simulink library "BESS_lib"  (Simulink 8.1)
settings: Solver=ode45  SolverMode=SingleTasking  StartTime=0.0  StopTime=10.0  RelTol=1e-3
undefined symbols (not defined in the file or in its folder): DiscIntNeverNeededParam, gcbh, sps_rtmsupport, Ts
libraries: simulink x25, powerlib x6, powerlib_meascontrol x4, powerlib_extras x3, simulink_extras x1, debounce_lib x1
(part 1 of 2)
settings Model: Creator=ch24070  LastModifiedBy=hptb1  CovMetricSettings=dwe  CovHtmlReporting=off  covSaveCumulativeToWorkspaceVar=off  CovSaveSingleToWorkspaceVar=off  CovExternalEMLEnable=on

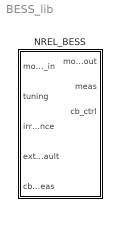
== system BESS_lib ==
  NREL_BESS : Subsystem  mask{InvType=ESS Inverter, Sn=250, Vn=480, b_Vdc_nom=1000, b_kWh=600, b_esr=0.1, r_I_max=3, Tc=Ts, MbusPrecInc=on, ExtTuningEna=on}
      mask prompts: InvType "Inverter type"; Sn "Nominal power [kVA]"; Vn "Nominal voltage ph-ph [V]"; b_Vdc_nom "Battery Vdc nominal [V]"; b_kWh "Battery capacity [kWh]"; b_esr "Battery ESR [Ohm]"; r_I_max "Max Current Ratio"; Tc "Control time step [s]"; MbusPrecInc "Increase power precision at Modbus interface (10x)"; ExtTuningEna "External tuning"
      mask init:
      | CFG.InvType = InvType;
      | CFG.Sn = Sn*1000;
      | CFG.Vn = Vn;
      | CFG.fn = 60;
      | CFG.r_I_max = r_I_max;
      | CFG.Tc = Tc;
      | 
      | if (MbusPrecInc == true)
      |     CFG.Prec = 10;
      | else
      |     CFG.Prec = 1;
      | end;
      | 
      | % get bess internal params (BP)
      | BP = BESS_init_mask(CFG);
      | 
      | 
      | dstr = 'Inverter data:\n';
      | dstr = [ dstr 'Sn=' num2str(Sn) 'kW\n'];
      | dstr = [ dstr 'Vn=' num2str(Vn/1000) 'kV\n'];
      | dstr = [ dstr 'In=' num2str(BP.In) 'A\n'];
      | dstr = [ dstr 'Imax=' num2str(BP.Imax) 'A\n'];
      mask TypeOptions InvType: PV Inverter | ESS Inverter
      mask Display: disp(dstr);

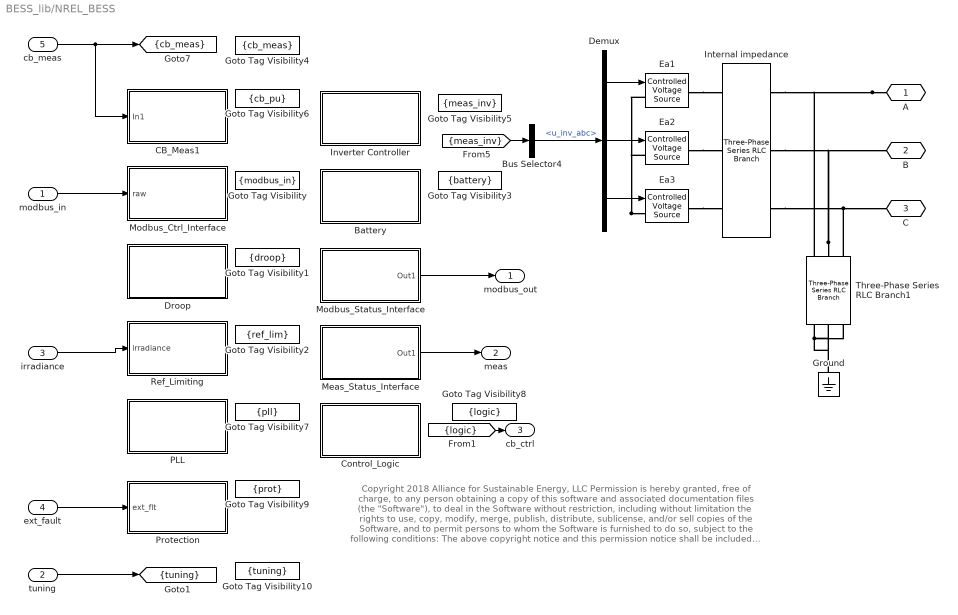
== system BESS_lib/NREL_BESS ==
  note: Copyright 2018 Alliance for Sustainable Energy, LLC
      |
      | Permission is hereby granted, free of charge, to any person obtaining a copy of this software
      | and associated documentation files (the "Software"), to deal in the Software without restriction,
      | including without limitation the rights to use, copy, modify, merge, publish, distribute, sublicense,
      | and/or sell copies of the Software, and to permit persons to whom the Software is furnished to do so,
      | subject to the following conditions:
      |
      | The above copyright notice and this permission notice shall be included in all copies or substantial portions of the Software.
      |
      | THE SOFTWARE IS PROVIDED "AS IS", WITHOUT WARRANTY OF ANY KIND, EXPRESS OR IMPLIED, INCLUDING
      | BUT NOT LIMITED TO THE WARRANTIES OF MERCHANTABILITY, FITNESS FOR A PARTICULAR PURPOSE AND
      | NONINFRINGEMENT. IN NO EVENT SHALL THE AUTHORS, THE COPYRIGHT HOLDERS, THE UNITED STATES,
      | THE UNITED STATES DEPARTMENT OF ENERGY, OR ANY OF THEIR EMPLOYEES BE LIABLE FOR ANY CLAIM,
      | DAMAGES OR OTHER LIABILITY, WHETHER IN AN ACTION OF CONTRACT, TORT OR OTHERWISE, ARISING FROM,
      | OUT OF OR IN CONNECTION WITH THE SOFTWARE OR THE USE OR OTHER DEALINGS IN THE SOFTWARE.
  modbus_in : Inport
  tuning : Inport  Port=2
  irradiance : Inport  Port=3
  ext_fault : Inport  Port=4
  cb_meas : Inport  Port=5
  Battery : Subsystem
  Bus Selector4 : BusSelector  OutputSignals=u_inv_abc
  CB_Meas1 : Subsystem
  Control_Logic : Subsystem
  Demux : Demux  Outputs=3
  Droop : Subsystem
  Ea1 : powerlib/Electrical Sources/Controlled Voltage Source  Initialize=off  Source_Type=DC  Amplitude=0  Phase=0  Frequency=0  Measurements=None
  Ea2 : powerlib/Electrical Sources/Controlled Voltage Source  Initialize=off  Source_Type=DC  Amplitude=0  Phase=0  Frequency=0  Measurements=None
  Ea3 : powerlib/Electrical Sources/Controlled Voltage Source  Initialize=off  Source_Type=DC  Amplitude=0  Phase=0  Frequency=0  Measurements=None
  Goto Tag Visibility : GotoTagVisibility  GotoTag=modbus_in
  Goto Tag Visibility1 : GotoTagVisibility  GotoTag=droop
  Goto Tag Visibility10 : GotoTagVisibility  GotoTag=tuning
  Goto Tag Visibility2 : GotoTagVisibility  GotoTag=ref_lim
  Goto Tag Visibility3 : GotoTagVisibility  GotoTag=battery
  Goto Tag Visibility4 : GotoTagVisibility  GotoTag=cb_meas
  Goto Tag Visibility5 : GotoTagVisibility  GotoTag=meas_inv
  Goto Tag Visibility6 : GotoTagVisibility  GotoTag=cb_pu
  Goto Tag Visibility7 : GotoTagVisibility  GotoTag=pll
  Goto Tag Visibility8 : GotoTagVisibility  GotoTag=logic
  Goto Tag Visibility9 : GotoTagVisibility  GotoTag=prot
  Ground : powerlib/Elements/Ground  LConnTagsString=a
  Internal impedance : powerlib/Elements/Three-Phase Series RLC Branch  LConnTagsString=A|B|C  RConnTagsString=A|B|C  BranchType=RL  Resistance=BP.R  Inductance=BP.L  Capacitance=1e-6  Measurements=None
  Inverter Controller : Subsystem
  Meas_Status_Interface : Subsystem
  Modbus_Ctrl_Interface : Subsystem
  Modbus_Status_Interface : Subsystem
  PLL : Subsystem
  Protection : Subsystem
  Ref_Limiting : Subsystem
  Three-Phase Series RLC Branch1 : powerlib/Elements/Three-Phase Series RLC Branch  LConnTagsString=A|B|C  RConnTagsString=A|B|C  BranchType=R  Resistance=10000  Inductance=1e-3  Capacitance=1000e-9  Measurements=None
  A : PMIOPort  Port=1  Side=Right
  B : PMIOPort  Port=2  Side=Right
  C : PMIOPort  Port=3  Side=Right
  modbus_out : Outport
  meas : Outport  Port=2
  cb_ctrl : Outport  Port=3
  tag scope: cb_meas=scoped, tuning=scoped
  wires:
  tuning/1 -> [tuning]
  ext_fault/1 -> Protection/1(ext_flt)
  Bus Selector4/1 -> Demux/1  "<u_inv_abc>"
  [meas_inv] -> Bus Selector4/1
  [logic] -> cb_ctrl/1
  Meas_Status_Interface/1(Out1) -> meas/1
  cb_meas/1 -> CB_Meas1/1(In1), [cb_meas]
  irradiance/1 -> Ref_Limiting/1(irradiance)
  Demux/1 -> Ea1/1
  Demux/2 -> Ea2/1
  Demux/3 -> Ea3/1
  Modbus_Status_Interface/1(Out1) -> modbus_out/1
  modbus_in/1 -> Modbus_Ctrl_Interface/1(raw)
  connections:
  Ea1/RConn1 -- Internal impedance/LConn1
  Ea2/RConn1 -- Internal impedance/LConn2
  Ea3/RConn1 -- Internal impedance/LConn3
  Ea3/LConn1 -- Ea2/LConn1 -- Ea1/LConn1
  A/RConn1 -- Internal impedance/RConn1 -- Three-Phase Series RLC Branch1/LConn1
  Internal impedance/RConn3 -- C/RConn1 -- Three-Phase Series RLC Branch1/LConn3
  Three-Phase Series RLC Branch1/LConn2 -- B/RConn1 -- Internal impedance/RConn2
  Three-Phase Series RLC Branch1/RConn1 -- Three-Phase Series RLC Branch1/RConn3 -- Three-Phase Series RLC Branch1/RConn2 -- Ground/LConn1

== system BESS_lib/NREL_BESS/Battery ==
  Battery : Subsystem  mask(Very simple battery model.){kWh=b_kWh, esr=b_esr, Vdc_nom=b_Vdc_nom}
      mask prompts: kWh "Capacity  (kWh)"; esr "Output Resistance (Ohms)"; Vdc_nom "Open Circuit Voltage"
      mask help: Model integrates charge and stops at the rated capacity. When charge is all removed the current drops to zero.
      mask Help: This model views the battery as a voltage source with a fixed equivalent series resistance and a perfect integrator for capacity.
  Bus Creator1 : BusCreator  Inputs=5
  Bus Selector1 : BusSelector  OutputSignals=batt_cap_div,batt_soc_rst
  Bus Selector4 : BusSelector  OutputSignals=relay_out.m.kw
  Compare To Constant : simulink/Logic and Bit Operations/Compare To Constant  relop===  const=1  OutDataTypeStr=boolean
  Compare To Constant1 : simulink/Logic and Bit Operations/Compare To Constant  relop===  const=-1  OutDataTypeStr=boolean
  Data Type Conversion : DataTypeConversion  OutDataTypeStr=double
  Data Type Conversion1 : DataTypeConversion  OutDataTypeStr=double
  Divide : Product  Inputs=*/
  Gain : Gain  Gain=100
  Gain2 : Gain  Gain=1000
  tag scope: battery=scoped
  wires:
  Bus Selector1/2 -> Battery/3(soc_rst)  "<batt_soc_rst>"
  Bus Selector1/1 -> Battery/2(cap_div)  "<batt_cap_div>"
  [tuning] -> Bus Selector1/1
  Gain2/1 -> Divide/1
  Bus Selector4/1 -> Gain2/1  "<kw>"
  Divide/1 -> Battery/1(Iout), Bus Creator1/5  "Idc"
  Battery/1(Vout) -> Bus Creator1/1, Divide/2  "Vdc"
  Gain/1 -> Bus Creator1/2  "SoC"
  Battery/2(Capacity) -> Gain/1
  Compare To Constant/1 -> Data Type Conversion/1
  Battery/3(Saturation) -> Compare To Constant1/1, Compare To Constant/1
  Compare To Constant1/1 -> Data Type Conversion1/1
  Bus Creator1/1 -> [battery]  "Battery"
  [cb_meas] -> Bus Selector4/1
  Data Type Conversion/1 -> Bus Creator1/3  "BattFull"
  Data Type Conversion1/1 -> Bus Creator1/4  "BattEmpty"

== system BESS_lib/NREL_BESS/CB_Meas1 ==
  In1 : Inport
  Bus Creator : BusCreator  Inputs=2
  Bus Selector : BusSelector  OutputSignals=cb_meas
  Bus Selector1 : BusSelector  OutputSignals=Vabc_line,Iabc
  Gain2 : Gain  Gain=1/BP.In/sqrt(2)
  Gain4 : Gain  Gain=1/(Vn*sqrt(2/3))
  tag scope: cb_pu=scoped
  wires:
  Bus Creator/1 -> [cb_pu]
  Gain2/1 -> Bus Creator/2  "iabc"
  Bus Selector1/2 -> Gain2/1  "<Iabc>"
  Gain4/1 -> Bus Creator/1  "vabc_line"
  Bus Selector1/1 -> Gain4/1  "<Vabc_line>"
  In1/1 -> Bus Selector/1
  Bus Selector/1 -> Bus Selector1/1  "<cb_meas>"

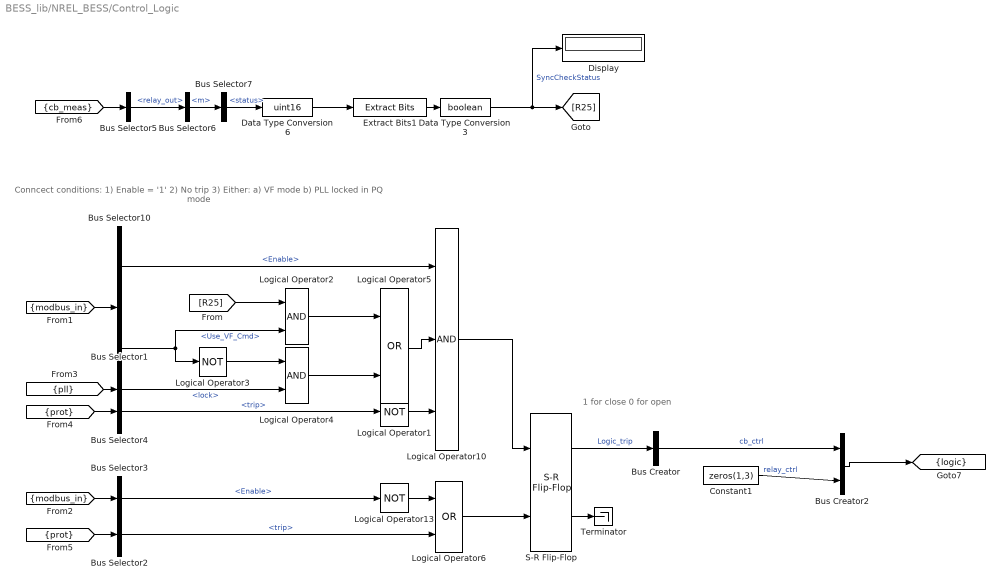
== system BESS_lib/NREL_BESS/Control_Logic ==
  note: 1 for close
      | 0 for open
  note: Conncect conditions:
      | 1) Enable = '1'
      | 2) No trip
      | 3) Either:
      | a) VF mode
      | b) PLL locked in PQ mode
  Bus Creator : BusCreator  Inputs=1
  Bus Creator2 : BusCreator  Inputs=2
  Bus Selector1 : BusSelector  OutputSignals=lock
  Bus Selector10 : BusSelector  OutputSignals=Control_Word.Enable,Control_Word.Use_VF_Cmd
  Bus Selector2 : BusSelector  OutputSignals=trip
  Bus Selector3 : BusSelector  OutputSignals=Control_Word.Enable
  Bus Selector4 : BusSelector  OutputSignals=trip
  Bus Selector5 : BusSelector  OutputSignals=relay_out
  Bus Selector6 : BusSelector  OutputSignals=m
  Bus Selector7 : BusSelector  OutputSignals=status
  Constant1 : Constant  Value=zeros(1,3)
  Data Type Conversion3 : DataTypeConversion  OutDataTypeStr=boolean
  Data Type Conversion6 : DataTypeConversion  OutDataTypeStr=uint16
  Display : Display
  Extract Bits1 : simulink/Logic and Bit Operations/Extract Bits  bitsToExtract=Range of bits  numBits=8  bitIdxRange=1  outScalingMode=Treat bit field as an integer
  Logical Operator1 : Logic  Operator=NOT  AllPortsSameDT=off  OutDataTypeStr=boolean
  Logical Operator10 : Logic  Inputs=3  AllPortsSameDT=off  OutDataTypeStr=boolean
  Logical Operator13 : Logic  Operator=NOT  AllPortsSameDT=off  OutDataTypeStr=boolean
  Logical Operator2 : Logic  AllPortsSameDT=off  OutDataTypeStr=boolean
  Logical Operator3 : Logic  Operator=NOT  AllPortsSameDT=off  OutDataTypeStr=boolean
  Logical Operator4 : Logic  AllPortsSameDT=off  OutDataTypeStr=boolean
  Logical Operator5 : Logic  Operator=OR  AllPortsSameDT=off  OutDataTypeStr=boolean
  Logical Operator6 : Logic  Operator=OR  AllPortsSameDT=off  OutDataTypeStr=boolean
  S-R Flip-Flop : simulink_extras/Flip Flops/S-R Flip-Flop  initial_condition=0
  Terminator : Terminator
  tag scope: logic=scoped
  wires:
  [R25] -> Logical Operator2/1
  Data Type Conversion3/1 -> [R25], Display/1  "SyncCheckStatus"
  Data Type Conversion6/1 -> Extract Bits1/1
  Extract Bits1/1 -> Data Type Conversion3/1
  Bus Selector7/1 -> Data Type Conversion6/1  "<status>"
  Bus Selector6/1 -> Bus Selector7/1  "<m>"
  Bus Selector5/1 -> Bus Selector6/1  "<relay_out>"
  [cb_meas] -> Bus Selector5/1
  Logical Operator2/1 -> Logical Operator5/1
  [prot] -> Bus Selector4/1
  Bus Selector4/1 -> Logical Operator1/1  "<trip>"
  [prot] -> Bus Selector2/1
  S-R Flip-Flop/2 -> Terminator/1
  Logical Operator13/1 -> Logical Operator6/1
  Bus Selector2/1 -> Logical Operator6/2  "<trip>"
  Logical Operator6/1 -> S-R Flip-Flop/2
  [modbus_in] -> Bus Selector3/1
  Bus Selector3/1 -> Logical Operator13/1  "<Enable>"
  Logical Operator1/1 -> Logical Operator10/3
  Logical Operator10/1 -> S-R Flip-Flop/1
  Logical Operator5/1 -> Logical Operator10/2
  Bus Selector1/1 -> Logical Operator4/2  "<lock>"
  Bus Selector10/2 -> Logical Operator3/1, Logical Operator2/2  "<Use_VF_Cmd>"
  [modbus_in] -> Bus Selector10/1
  Bus Selector10/1 -> Logical Operator10/1  "<Enable>"
  Constant1/1 -> Bus Creator2/2  "relay_ctrl"
  Bus Creator2/1 -> [logic]
  Bus Creator/1 -> Bus Creator2/1  "cb_ctrl"
  Logical Operator3/1 -> Logical Operator4/1
  [pll] -> Bus Selector1/1
  S-R Flip-Flop/1 -> Bus Creator/1  "Logic_trip"
  Logical Operator4/1 -> Logical Operator5/2

== system BESS_lib/NREL_BESS/Droop ==
  Bus Selector1 : BusSelector  OutputSignals=relay_out
  Bus Selector3 : BusSelector  OutputSignals=m.Hz,m.Va_rms,m.kw,m.kvar  OutputAsBus=on
  Bus Selector9 : BusSelector  OutputSignals=f_cmd,v_cmd,p_cmd,q_cmd  OutputAsBus=on
  Constant : Constant  Value=[0 0]
  Divide1 : Product  Inputs=*/
  Droop : Subsystem
  ExtractCoefs : Subsystem
  Mux1 : Mux  Inputs=2
  ScalingFactors1 : Constant  Value=[60 Vn/sqrt(3) [1 1]*Sn]
  Selector1 : Selector  InputPortWidth=4  IndexOptions=Index vector (dialog)  Indices=[1 2]  OutputSizes=1
  Sum1 : Sum  Inputs=-+|
  Sum2 : Sum  Inputs=++|
  tag scope: droop=scoped
  wires:
  ExtractCoefs/1(Out1) -> Droop/2(droop)
  [modbus_in] -> ExtractCoefs/1(In1)
  Bus Selector3/1 -> Divide1/1
  Bus Selector1/1 -> Bus Selector3/1  "<relay_out>"
  [cb_meas] -> Bus Selector1/1
  Bus Selector9/1 -> Selector1/1, Sum2/2
  [modbus_in] -> Bus Selector9/1
  Droop/1(dFvpq_out) -> Sum2/1
  Sum1/1 -> Droop/1(dfvpq)
  Selector1/1 -> Mux1/1
  Mux1/1 -> Sum1/2
  Constant/1 -> Mux1/2
  ScalingFactors1/1 -> Divide1/2
  Divide1/1 -> Sum1/1
  Sum2/1 -> [droop]

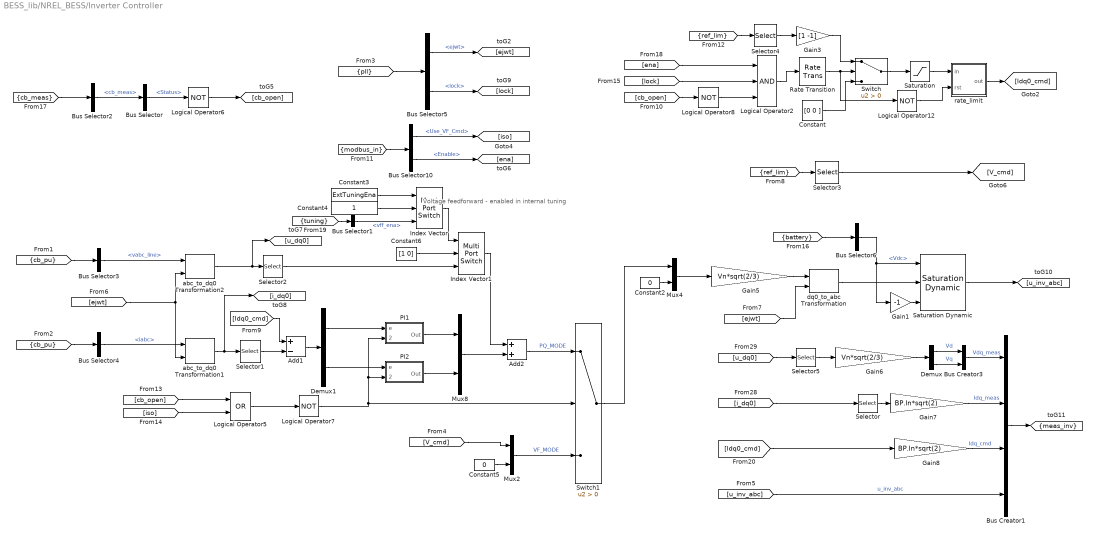
== system BESS_lib/NREL_BESS/Inverter Controller ==
  note: Voltage feedforward
      | - enabled in internal tuning
  Add1 : Sum  Inputs=+-
  Add2 : Sum
  Bus Creator1 : BusCreator
  Bus Creator3 : BusCreator  Inputs=2
  Bus Selector : BusSelector  OutputSignals=Status
  Bus Selector1 : BusSelector  OutputSignals=vff_ena
  Bus Selector10 : BusSelector  OutputSignals=Control_Word.Use_VF_Cmd,Control_Word.Enable
  Bus Selector2 : BusSelector  OutputSignals=cb_meas
  Bus Selector3 : BusSelector  OutputSignals=vabc_line
  Bus Selector4 : BusSelector  OutputSignals=iabc
  Bus Selector5 : BusSelector  OutputSignals=ejwt,lock
  Bus Selector6 : BusSelector  OutputSignals=Vdc
  Constant : Constant  Value=[0 0 ]
  Constant2 : Constant  Value=0
  Constant3 : Constant  Value=ExtTuningEna
  Constant4 : Constant
  Constant5 : Constant  Value=0
  Constant6 : Constant  Value=[1 0]
  Demux : Demux  Outputs=2
  Demux1 : Demux  Outputs=2
  Gain1 : Gain  Gain=-1
  Gain3 : Gain  Gain=[1 -1]
  Gain5 : Gain  Gain=Vn*sqrt(2/3)
  Gain6 : Gain  Gain=Vn*sqrt(2/3)
  Gain7 : Gain  Gain=BP.In*sqrt(2)
  Gain8 : Gain  Gain=BP.In*sqrt(2)
  Index Vector : MultiPortSwitch  DataPortOrder=Zero-based contiguous  Inputs=2  zeroidx=on
  Index Vector1 : MultiPortSwitch  DataPortOrder=Zero-based contiguous  Inputs=2  zeroidx=on
  Logical Operator{6..8,12} (4 alike) : Logic  Operator=NOT  AllPortsSameDT=off  OutDataTypeStr=boolean
  Logical Operator2 : Logic  Inputs=3  AllPortsSameDT=off  OutDataTypeStr=boolean
  Logical Operator5 : Logic  Operator=OR  AllPortsSameDT=off  OutDataTypeStr=boolean
  Mux2 : Mux  Inputs=2
  Mux4 : Mux  Inputs=[2 1]
  Mux8 : Mux  Inputs=2
  PI1 : Subsystem  mask{Kp=2, Ti=0.6e-3, Ts=Ts, D=0, Iup=1, Idown=-1, PIup=1, PIdown=-1, Int_init=0, Enable_zero_val=0}
      mask prompts: Kp "Proportional gain Kp"; Ti "Integral doubling-time Ti [s]"; Ts "Sample time [s]"; D "Derivative Gain"; Iup "Integral upper saturation limit"; Idown "Integral lower saturation limit"; PIup "PI output upper saturation limit"; PIdown "PI output lower saturation limit"; Int_init "Integral initial value"; Enable_zero_val "Output value when Enable=0"
      mask help: PID controller integral is in enable state when Enable signal value equals 1. If Enable state equals zero the PID output also equals zero.
  PI2 : Subsystem  mask{Kp=2, Ti=0.6e-3, Ts=Ts, D=0, Iup=1, Idown=-1, PIup=1, PIdown=-1, Int_init=0, Enable_zero_val=0}
      mask prompts: Kp "Proportional gain Kp"; Ti "Integral doubling-time Ti [s]"; Ts "Sample time [s]"; D "Derivative Gain"; Iup "Integral upper saturation limit"; Idown "Integral lower saturation limit"; PIup "PI output upper saturation limit"; PIdown "PI output lower saturation limit"; Int_init "Integral initial value"; Enable_zero_val "Output value when Enable=0"
      mask help: PID controller integral is in enable state when Enable signal value equals 1. If Enable state equals zero the PID output also equals zero.
  Rate Transition : RateTransition  OutPortSampleTime=Tc
  Saturation : Saturate  UpperLimit=BP.Imax*sqrt(2)  LowerLimit=-BP.Imax*sqrt(2)
  Saturation Dynamic : simulink/Discontinuities/Saturation Dynamic  OutMin=[]  OutMax=[]  OutDataTypeStr=Inherit: Same as second input  OutDataType=fixdt(1, 16)  OutScaling=2^-10  DoSatur=off
  Selector{,1..2,5} (4 alike) : Selector  InputPortWidth=3  IndexOptions=Index vector (dialog)  Indices=[1 2]  OutputSizes=1
  Selector3 : Selector  InputPortWidth=4  IndexOptions=Index vector (dialog)  Indices=2  OutputSizes=1
  Selector4 : Selector  InputPortWidth=4  IndexOptions=Index vector (dialog)  Indices=[3 4]  OutputSizes=1
  Switch : Switch  Criteria=u2 > Threshold
  Switch1 : Switch  Criteria=u2 > Threshold
  abc_to_dq0 Transformation1 : powerlib_extras/Measurements/abc_to_dq0 Transformation
  abc_to_dq0 Transformation2 : powerlib_extras/Measurements/abc_to_dq0 Transformation
  dq0_to_abc Transformation : powerlib_extras/Measurements/dq0_to_abc Transformation
  rate_limit : Subsystem
  tag scope: meas_inv=scoped
  wires:
  Constant6/1 -> Index Vector1/2
  Selector2/1 -> Index Vector1/3
  Index Vector/1 -> Index Vector1/1
  Constant4/1 -> Index Vector/2
  Bus Selector1/1 -> Index Vector/3  "<vff_ena>"
  [tuning] -> Bus Selector1/1
  Constant3/1 -> Index Vector/1
  Bus Selector6/1 -> Gain1/1, Saturation Dynamic/1  "<Vdc>"
  [battery] -> Bus Selector6/1
  Bus Selector10/1 -> [iso]  "<Use_VF_Cmd>"
  [modbus_in] -> Bus Selector10/1
  Bus Selector10/2 -> [ena]  "<Enable>"
  [ref_lim] -> Selector3/1
  [ref_lim] -> Selector4/1
  [u_inv_abc] -> Bus Creator1/4  "u_inv_abc"
  Bus Selector5/2 -> [lock]  "<lock>"
  Bus Selector5/1 -> [ejwt]  "<ejwt>"
  [pll] -> Bus Selector5/1
  [cb_pu] -> Bus Selector4/1
  [cb_pu] -> Bus Selector3/1
  Gain3/1 -> Switch/1
  Bus Selector2/1 -> Bus Selector/1  "<cb_meas>"
  Demux/2 -> Bus Creator3/2  "Vq"
  Demux/1 -> Bus Creator3/1  "Vd"
  Gain6/1 -> Demux/1
  Bus Creator3/1 -> Bus Creator1/1  "Vdq_meas"
  Gain8/1 -> Bus Creator1/3  "Idq_cmd"
  Gain7/1 -> Bus Creator1/2  "Idq_meas"
  Gain5/1 -> dq0_to_abc Transformation/1
  Bus Selector3/1 -> abc_to_dq0 Transformation2/1  "<vabc_line>"
  Bus Selector4/1 -> abc_to_dq0 Transformation1/1  "<iabc>"
  Gain1/1 -> Saturation Dynamic/3
  Saturation Dynamic/1 -> [u_inv_abc]
  Logical Operator12/1 -> rate_limit/2(rst)
  rate_limit/1(out) -> [Idq0_cmd]
  Selector5/1 -> Gain6/1
  Constant2/1 -> Mux4/2
  Mux4/1 -> Gain5/1
  Switch1/1 -> Mux4/1
  Index Vector1/1 -> Add2/1
  Selector1/1 -> Add1/2
  [i_dq0] -> Selector/1
  Bus Creator1/1 -> [meas_inv]
  [u_dq0] -> Selector5/1
  [Idq0_cmd] -> Gain8/1
  Selector/1 -> Gain7/1
  Selector3/1 -> [V_cmd]
  [ena] -> Logical Operator2/1
  Add2/1 -> Switch1/1  "PQ_MODE"
  Mux8/1 -> Add2/2
  abc_to_dq0 Transformation2/1 -> Selector2/1, [u_dq0]
  [lock] -> Logical Operator2/2
  [Idq0_cmd] -> Add1/1
  Saturation/1 -> rate_limit/1(in)
  Logical Operator8/1 -> Logical Operator2/3
  [cb_open] -> Logical Operator8/1
  [cb_open] -> Logical Operator5/1
  Logical Operator6/1 -> [cb_open]
  Bus Selector/1 -> Logical Operator6/1  "<Status>"
  [iso] -> Logical Operator5/2
  Logical Operator7/1 -> PI1/2(Enable), PI2/2(Enable), Switch1/2
  Logical Operator2/1 -> Rate Transition/1
  Constant/1 -> Switch/3
  Switch/1 -> Saturation/1
  Rate Transition/1 -> Switch/2, Logical Operator12/1
  Add1/1 -> Demux1/1
  Demux1/2 -> PI2/1(e)
  Demux1/1 -> PI1/1(e)
  Mux2/1 -> Switch1/3  "VF_MODE"
  Constant5/1 -> Mux2/2
  [V_cmd] -> Mux2/1
  Logical Operator5/1 -> Logical Operator7/1
  PI2/1(Out) -> Mux8/2
  PI1/1(Out) -> Mux8/1
  [ejwt] -> abc_to_dq0 Transformation2/2, abc_to_dq0 Transformation1/2
  [ejwt] -> dq0_to_abc Transformation/2
  Selector4/1 -> Gain3/1
  abc_to_dq0 Transformation1/1 -> Selector1/1, [i_dq0]
  [cb_meas] -> Bus Selector2/1
  dq0_to_abc Transformation/1 -> Saturation Dynamic/2

== system BESS_lib/NREL_BESS/Meas_Status_Interface ==
  Bus Creator4 : BusCreator  Inputs=6
  Bus Selector1 : BusSelector  OutputSignals=cb_ctrl.Logic_trip
  Bus Selector2 : BusSelector  OutputSignals=raw
  Bus Selector4 : BusSelector  OutputSignals=status,flt_word  OutputAsBus=on
  Data Type Conversion : DataTypeConversion  OutDataTypeStr=double
  Gain : Gain  Gain=[1 8]
  Sum : Sum  Inputs=+
  Out1 : Outport
  wires:
  Bus Selector2/1 -> Bus Creator4/6  "<raw>"
  [modbus_in] -> Bus Selector2/1
  Data Type Conversion/1 -> Bus Creator4/5  "Logic_trip"
  Bus Selector1/1 -> Data Type Conversion/1  "<Logic_trip>"
  [logic] -> Bus Selector1/1
  Sum/1 -> Bus Creator4/4  "status_word"
  Gain/1 -> Sum/1
  Bus Selector4/1 -> Gain/1
  [prot] -> Bus Selector4/1
  [meas_inv] -> Bus Creator4/1  "Inverter"
  [cb_meas] -> Bus Creator4/2  "CB_meas"
  Bus Creator4/1 -> Out1/1
  [battery] -> Bus Creator4/3  "Battery"

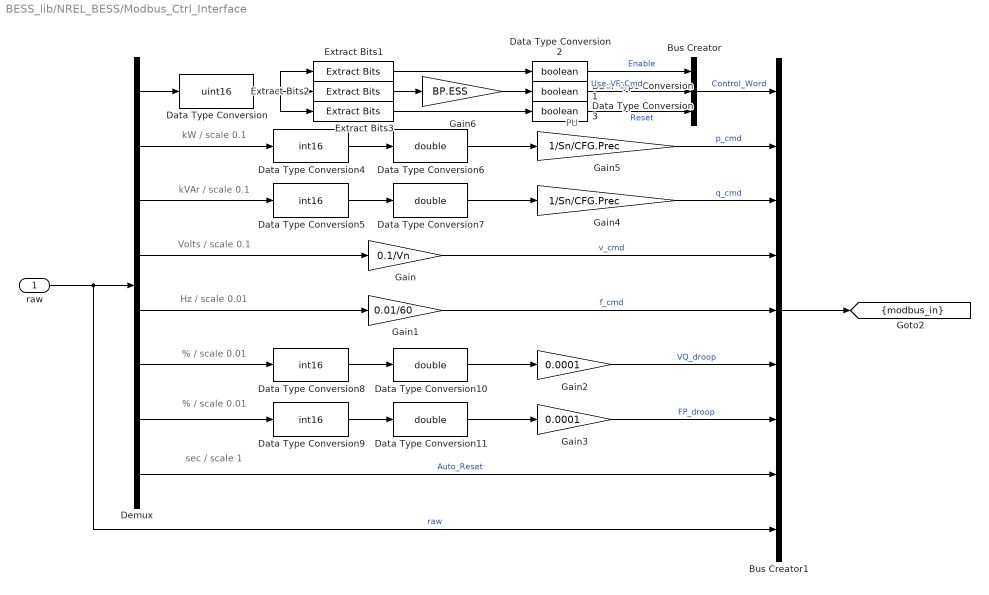
== system BESS_lib/NREL_BESS/Modbus_Ctrl_Interface ==
  note: sec / scale 1
  note: % / scale 0.01
  note: % / scale 0.01
  note: Hz / scale 0.01
  note: Volts / scale 0.1
  note: kVAr / scale 0.1
  note: PU
  note: kW / scale 0.1
  raw : Inport
  Bus Creator : BusCreator  Inputs=3
  Bus Creator1 : BusCreator  Inputs=9
  Data Type Conversion : DataTypeConversion  OutDataTypeStr=uint16
  Data Type Conversion1 : DataTypeConversion  OutDataTypeStr=boolean
  Data Type Conversion{6..7,10..11} (4 alike) : DataTypeConversion  OutDataTypeStr=double
  Data Type Conversion2 : DataTypeConversion  OutDataTypeStr=boolean
  Data Type Conversion3 : DataTypeConversion  OutDataTypeStr=boolean
  Data Type Conversion{4..5,8..9} (4 alike) : DataTypeConversion  OutDataTypeStr=int16
  Demux : Demux  Outputs=8
  Extract Bits1 : simulink/Logic and Bit Operations/Extract Bits  bitsToExtract=Range of bits  numBits=8  bitIdxRange=[0]  outScalingMode=Treat bit field as an integer
  Extract Bits2 : simulink/Logic and Bit Operations/Extract Bits  bitsToExtract=Range of bits  numBits=8  bitIdxRange=[1]  outScalingMode=Treat bit field as an integer
  Extract Bits3 : simulink/Logic and Bit Operations/Extract Bits  bitsToExtract=Range of bits  numBits=8  bitIdxRange=[2]  outScalingMode=Treat bit field as an integer
  Gain : Gain  Gain=0.1/Vn
  Gain1 : Gain  Gain=0.01/60
  Gain2 : Gain  Gain=0.0001
  Gain3 : Gain  Gain=0.0001
  Gain4 : Gain  Gain=1/Sn/CFG.Prec
  Gain5 : Gain  Gain=1/Sn/CFG.Prec
  Gain6 : Gain  Gain=BP.ESS
  tag scope: modbus_in=scoped
  wires:
  raw/1 -> Demux/1, Bus Creator1/9  "raw"
  Data Type Conversion11/1 -> Gain3/1
  Data Type Conversion10/1 -> Gain2/1
  Data Type Conversion9/1 -> Data Type Conversion11/1
  Data Type Conversion8/1 -> Data Type Conversion10/1
  Gain6/1 -> Data Type Conversion1/1
  Data Type Conversion7/1 -> Gain4/1
  Data Type Conversion6/1 -> Gain5/1
  Data Type Conversion5/1 -> Data Type Conversion7/1
  Data Type Conversion4/1 -> Data Type Conversion6/1
  Gain5/1 -> Bus Creator1/2  "p_cmd"
  Gain4/1 -> Bus Creator1/3  "q_cmd"
  Demux/2 -> Data Type Conversion4/1
  Data Type Conversion3/1 -> Bus Creator/3  "Reset"
  Data Type Conversion1/1 -> Bus Creator/2  "Use_VF_Cmd"
  Data Type Conversion2/1 -> Bus Creator/1  "Enable"
  Bus Creator1/1 -> [modbus_in]
  Demux/8 -> Bus Creator1/8  "Auto_Reset"
  Gain3/1 -> Bus Creator1/7  "FP_droop"
  Demux/7 -> Data Type Conversion9/1
  Gain2/1 -> Bus Creator1/6  "VQ_droop"
  Demux/6 -> Data Type Conversion8/1
  Gain1/1 -> Bus Creator1/5  "f_cmd"
  Demux/5 -> Gain1/1
  Gain/1 -> Bus Creator1/4  "v_cmd"
  Demux/4 -> Gain/1
  Demux/3 -> Data Type Conversion5/1
  Bus Creator/1 -> Bus Creator1/1  "Control_Word"
  Extract Bits3/1 -> Data Type Conversion3/1
  Extract Bits2/1 -> Gain6/1
  Extract Bits1/1 -> Data Type Conversion2/1
  Data Type Conversion/1 -> Extract Bits1/1, Extract Bits2/1, Extract Bits3/1
  Demux/1 -> Data Type Conversion/1

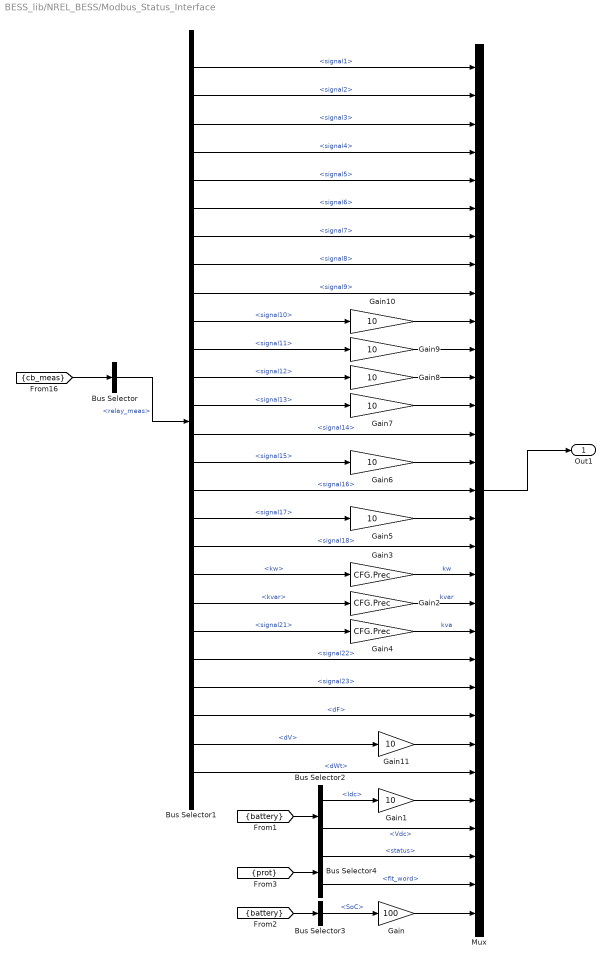
== system BESS_lib/NREL_BESS/Modbus_Status_Interface ==
  Bus Selector : BusSelector  OutputSignals=relay_meas
  Bus Selector1 : BusSelector  OutputSignals=signal1,signal2,signal3,signal4,signal5,signal6,signal7,signal8,signal9,signal10,signal11,signal12,signal13,signal14,signal15,signal16,signal17,signal18,kw,kvar,signal21,signal22,signal23,dF,dV,dWt
  Bus Selector2 : BusSelector  OutputSignals=Idc,Vdc
  Bus Selector3 : BusSelector  OutputSignals=SoC
  Bus Selector4 : BusSelector  OutputSignals=status,flt_word
  Gain : Gain  Gain=100
  Gain{1,5..11} (8 alike) : Gain  Gain=10
  Gain2 : Gain  Gain=CFG.Prec
  Gain3 : Gain  Gain=CFG.Prec
  Gain4 : Gain  Gain=CFG.Prec
  Mux : Mux  Inputs=31
  Out1 : Outport
  wires:
  Gain11/1 -> Mux/25
  Bus Selector1/26 -> Mux/26  "<dWt>"
  Bus Selector1/25 -> Gain11/1  "<dV>"
  Bus Selector1/24 -> Mux/24  "<dF>"
  Gain10/1 -> Mux/10
  Gain9/1 -> Mux/11
  Gain8/1 -> Mux/12
  Gain7/1 -> Mux/13
  Gain6/1 -> Mux/15
  Gain5/1 -> Mux/17
  Gain3/1 -> Mux/19  "kw"
  Gain2/1 -> Mux/20  "kvar"
  Gain4/1 -> Mux/21  "kva"
  Bus Selector4/1 -> Mux/29  "<status>"
  [prot] -> Bus Selector4/1
  Gain1/1 -> Mux/27
  Gain/1 -> Mux/31
  Bus Selector4/2 -> Mux/30  "<flt_word>"
  Bus Selector3/1 -> Gain/1  "<SoC>"
  [battery] -> Bus Selector3/1
  Bus Selector2/1 -> Gain1/1  "<Idc>"
  Bus Selector2/2 -> Mux/28  "<Vdc>"
  [battery] -> Bus Selector2/1
  Bus Selector1/23 -> Mux/23  "<signal23>"
  Bus Selector1/22 -> Mux/22  "<signal22>"
  Bus Selector1/21 -> Gain4/1  "<signal21>"
  Bus Selector1/20 -> Gain2/1  "<kvar>"
  Bus Selector1/19 -> Gain3/1  "<kw>"
  Bus Selector1/18 -> Mux/18  "<signal18>"
  Bus Selector1/17 -> Gain5/1  "<signal17>"
  Bus Selector1/16 -> Mux/16  "<signal16>"
  Bus Selector1/15 -> Gain6/1  "<signal15>"
  Bus Selector1/14 -> Mux/14  "<signal14>"
  Bus Selector1/13 -> Gain7/1  "<signal13>"
  Bus Selector1/12 -> Gain8/1  "<signal12>"
  Bus Selector1/11 -> Gain9/1  "<signal11>"
  Bus Selector1/10 -> Gain10/1  "<signal10>"
  Bus Selector1/9 -> Mux/9  "<signal9>"
  Bus Selector1/8 -> Mux/8  "<signal8>"
  Bus Selector1/7 -> Mux/7  "<signal7>"
  Bus Selector1/6 -> Mux/6  "<signal6>"
  Bus Selector1/5 -> Mux/5  "<signal5>"
  Bus Selector1/4 -> Mux/4  "<signal4>"
  Bus Selector1/3 -> Mux/3  "<signal3>"
  Bus Selector1/2 -> Mux/2  "<signal2>"
  Bus Selector1/1 -> Mux/1  "<signal1>"
  Bus Selector/1 -> Bus Selector1/1  "<relay_meas>"
  Mux/1 -> Out1/1
  [cb_meas] -> Bus Selector/1

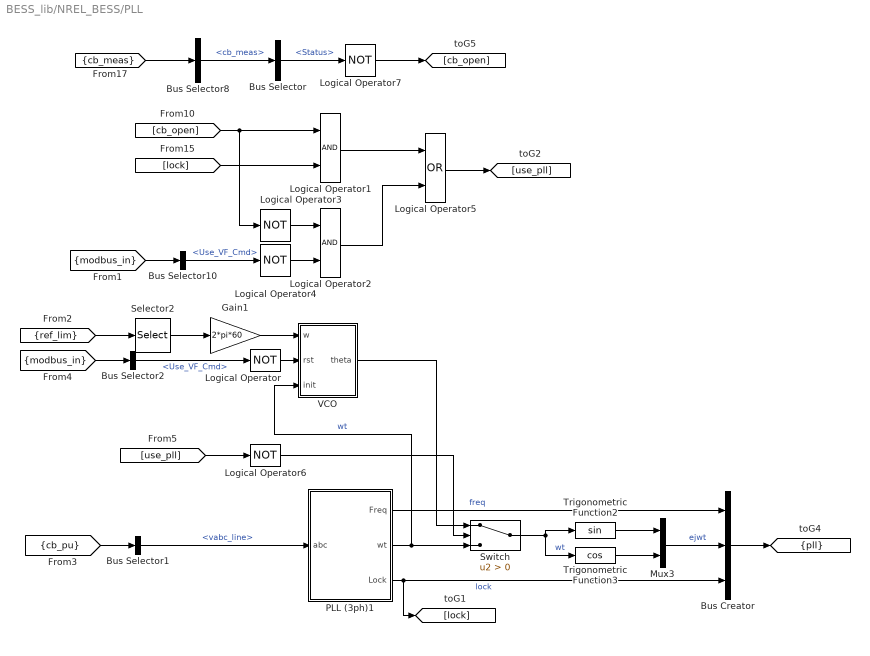
== system BESS_lib/NREL_BESS/PLL ==
  Bus Creator : BusCreator  Inputs=3
  Bus Selector : BusSelector  OutputSignals=Status
  Bus Selector1 : BusSelector  OutputSignals=vabc_line
  Bus Selector10 : BusSelector  OutputSignals=Control_Word.Use_VF_Cmd
  Bus Selector2 : BusSelector  OutputSignals=Control_Word.Use_VF_Cmd
  Bus Selector8 : BusSelector  OutputSignals=cb_meas
  Gain1 : Gain  Gain=2*pi*60  SaturateOnIntegerOverflow=on  OutDataTypeStr=Inherit: Same as input  ParamDataTypeStr=Inherit: Same as input
  Logical Operator{,3..4,6..7} (5 alike) : Logic  Operator=NOT  AllPortsSameDT=off  OutDataTypeStr=boolean
  Logical Operator1 : Logic  AllPortsSameDT=off  OutDataTypeStr=boolean
  Logical Operator2 : Logic  AllPortsSameDT=off  OutDataTypeStr=boolean
  Logical Operator5 : Logic  Operator=OR  AllPortsSameDT=off  OutDataTypeStr=boolean
  Mux3 : Mux  Inputs=2
  PLL (3ph)1 : Subsystem  DialogController=POWERSYS.PowerSysDialog  LoadFcn=sps_rtmsupport('LoadFcn', gcbh);  StartFcn=sps_rtmsupport('StartFcn', gcbh);  StopFcn=sps_rtmsupport('StopFcn', gcbh);  mask(PLL (3ph)){Flim=[55 66], Par_Init=[0, 60], ParK=[180, 3200, 1], TcD=Tc, MaxRateChangeFreq=12, FilterCutOffFreq=25, Ts=Tc, AGC=off}
      mask prompts: Flim "Minimum frequency (Hz):"; Par_Init "Initial inputs [ Phase (degrees), Frequency (Hz) ]:"; ParK "Regulator gains [ Kp, Ki, Kd ]:"; TcD "Time constant for derivative action (s):"; MaxRateChangeFreq "Maximum rate of change of frequency (Hz/s):"; FilterCutOffFreq "Filter cut-off frequency for frequency measurement (Hz):"; Ts "Sample time:"; AGC "Enable automatic gain control"
      mask help:
      | This Phase Locked Loop (PLL) system can be used  to synchronize on a set of variable frequency, three-phase sinusoidal signals. If the Automatic Gain Control is enabled, the input (phase error) of the PLL regulator is scaled according to the input signals magnitude.
      |
      | For optimal performance, set regulator gains [ Kp Ki  Kd ] = [ 180  3200  1 ] and check the Enable Automatic Gain Control parameter.
      |
      | Input : Vector containing the normalized three-phase signals [Va Vb Vc]
      | Output 1:  Measured frequency (Hz) = w/(2pi)
      | Output 2:  Ramp w.t varying between  0 and 2*pi, synchronized on zero crossings of the fundamental (positive-sequence) of phase A.
      mask init:
      | %block=gcb;
      | %[WantBlockChoice,Ts,sps] = powericon('PLL3phInit',block,Fmin,Par_Init,ParK,TcD, MaxRateChangeFreq, FilterCutOffFreq, AGC,Ts);
      | %powericon('SetInternalModels','set',block,WantBlockChoice);
      settings: CopyFcn=sps_rtmsupport('CopyFcn', gcbh);  DeleteFcn=sps_rtmsupport('DeleteFcn', gcbh);  UndoDeleteFcn=sps_rtmsupport('UndoDeleteFcn', gcbh);  ModelCloseFcn=sps_rtmsupport('ModelCloseFcn', gcbh);  PreSaveFcn=sps_rtmsupport('PreSaveFcn', gcbh);  PostSaveFcn=sps_rtmsupport('PostSaveFcn', gcbh);  NameChangeFcn=sps_rtmsupport('NameChangeFcn', gcbh);  PreCopyFcn=sps_rtmsupport('PreCopyFcn', gcbh);  CloseFcn=sps_rtmsupport('CloseFcn', gcbh);  PreDeleteFcn=sps_rtmsupport('PreDeleteFcn', gcbh);
      settings: OpenFcn=|
      | power_openblockproxy();
      | sps_rtmsupport('OpenFcn', gcbh, [8]);
      mask Help: helpview(psbhelp);
  Selector2 : Selector  InputPortWidth=4  IndexOptions=Index vector (dialog)  Indices=[1]  OutputSizes=1
  Switch : Switch  Criteria=u2 > Threshold
  Trigonometric Function2 : Trigonometry
  Trigonometric Function3 : Trigonometry  Operator=cos
  VCO : Subsystem
  tag scope: pll=scoped
  wires:
  Logical Operator6/1 -> Switch/2
  Logical Operator5/1 -> [use_pll]
  Logical Operator2/1 -> Logical Operator5/2
  Logical Operator4/1 -> Logical Operator2/2
  Logical Operator3/1 -> Logical Operator2/1
  Bus Selector10/1 -> Logical Operator4/1  "<Use_VF_Cmd>"
  Bus Selector2/1 -> Logical Operator/1  "<Use_VF_Cmd>"
  [modbus_in] -> Bus Selector2/1
  Logical Operator1/1 -> Logical Operator5/1
  [lock] -> Logical Operator1/2
  [cb_open] -> Logical Operator1/1, Logical Operator3/1
  Bus Selector8/1 -> Bus Selector/1  "<cb_meas>"
  Logical Operator7/1 -> [cb_open]
  Bus Selector/1 -> Logical Operator7/1  "<Status>"
  [cb_meas] -> Bus Selector8/1
  Logical Operator/1 -> VCO/2(rst)
  PLL (3ph)1/2(wt) -> Switch/3, VCO/3(init)  "wt"
  VCO/1(theta) -> Switch/1
  Gain1/1 -> VCO/1(w)
  [cb_pu] -> Bus Selector1/1
  [ref_lim] -> Selector2/1
  [use_pll] -> Logical Operator6/1
  [modbus_in] -> Bus Selector10/1
  Bus Creator/1 -> [pll]
  Selector2/1 -> Gain1/1
  PLL (3ph)1/1(Freq) -> Bus Creator/1  "freq"
  PLL (3ph)1/3(Lock) -> Bus Creator/3, [lock]  "lock"
  Bus Selector1/1 -> PLL (3ph)1/1(abc)  "<vabc_line>"
  Trigonometric Function3/1 -> Mux3/2
  Trigonometric Function2/1 -> Mux3/1
  Switch/1 -> Trigonometric Function3/1, Trigonometric Function2/1  "wt"
  Mux3/1 -> Bus Creator/2  "ejwt"

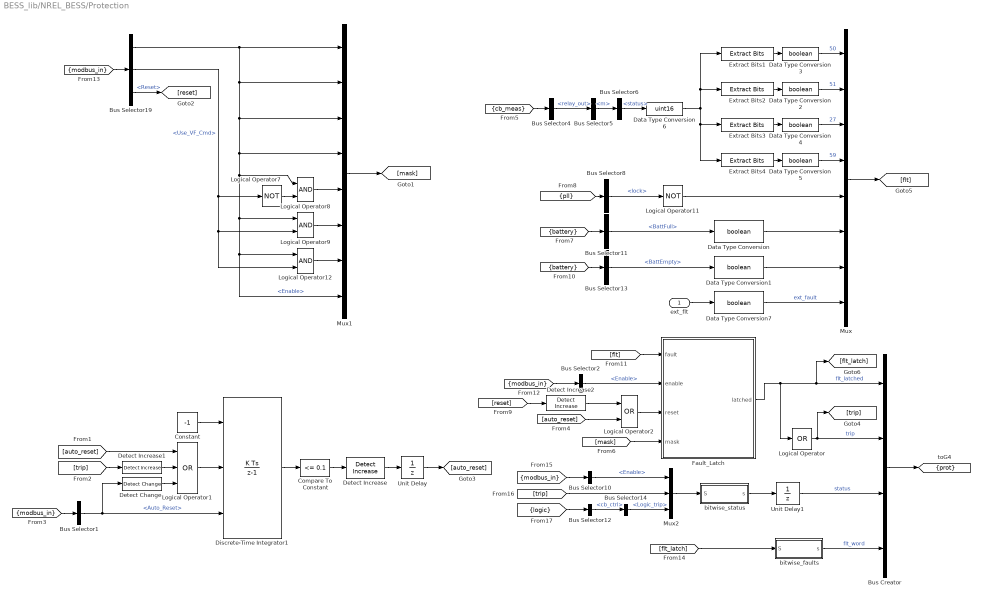
== system BESS_lib/NREL_BESS/Protection ==
  ext_flt : Inport
  Bus Creator : BusCreator
  Bus Selector1 : BusSelector  OutputSignals=Auto_Reset
  Bus Selector10 : BusSelector  OutputSignals=Control_Word.Enable
  Bus Selector11 : BusSelector  OutputSignals=BattFull
  Bus Selector12 : BusSelector  OutputSignals=cb_ctrl
  Bus Selector13 : BusSelector  OutputSignals=BattEmpty
  Bus Selector14 : BusSelector  OutputSignals=Logic_trip
  Bus Selector19 : BusSelector  OutputSignals=Control_Word.Enable,Control_Word.Use_VF_Cmd,Control_Word.Reset
  Bus Selector2 : BusSelector  OutputSignals=Control_Word.Enable
  Bus Selector4 : BusSelector  OutputSignals=relay_out
  Bus Selector5 : BusSelector  OutputSignals=m
  Bus Selector6 : BusSelector  OutputSignals=status
  Bus Selector8 : BusSelector  OutputSignals=lock
  Compare To Constant : simulink/Logic and Bit Operations/Compare To Constant  relop=<=  const=0.1  OutDataTypeStr=boolean
  Constant : Constant  Value=-1
  Data Type Conversion{,1..5,7} (7 alike) : DataTypeConversion  OutDataTypeStr=boolean
  Data Type Conversion6 : DataTypeConversion  OutDataTypeStr=uint16
  Detect Change : simulink/Logic and Bit Operations/Detect Change  vinit=0  InputProcessing=Inherited  OutDataTypeStr=boolean
  Detect Increase : simulink/Logic and Bit Operations/Detect Increase  vinit=0.0  InputProcessing=Inherited  OutDataTypeStr=boolean
  Detect Increase1 : simulink/Logic and Bit Operations/Detect Increase  vinit=0.0  InputProcessing=Inherited  OutDataTypeStr=boolean
  Detect Increase2 : simulink/Logic and Bit Operations/Detect Increase  vinit=0.0  InputProcessing=Inherited  OutDataTypeStr=boolean
  Discrete-Time Integrator1 : DiscreteIntegrator  ExternalReset=rising  InitialConditionSource=external  SampleTime=Ts  LimitOutput=on  LowerSaturationLimit=0  ICPrevOutput=DiscIntNeverNeededParam  ICPrevScaledInput=DiscIntNeverNeededParam
  Extract Bits1 : simulink/Logic and Bit Operations/Extract Bits  bitsToExtract=Range of bits  numBits=8  bitIdxRange=7  outScalingMode=Treat bit field as an integer
  Extract Bits2 : simulink/Logic and Bit Operations/Extract Bits  bitsToExtract=Range of bits  numBits=8  bitIdxRange=8  outScalingMode=Treat bit field as an integer
  Extract Bits3 : simulink/Logic and Bit Operations/Extract Bits  bitsToExtract=Range of bits  numBits=8  bitIdxRange=9  outScalingMode=Treat bit field as an integer
  Extract Bits4 : simulink/Logic and Bit Operations/Extract Bits  bitsToExtract=Range of bits  numBits=8  bitIdxRange=10  outScalingMode=Treat bit field as an integer
  Fault_Latch : Subsystem
  Logical Operator : Logic  Operator=OR  Inputs=1  AllPortsSameDT=off  OutDataTypeStr=boolean
  Logical Operator1 : Logic  Operator=OR  Inputs=3  AllPortsSameDT=off  OutDataTypeStr=boolean
  Logical Operator11 : Logic  Operator=NOT  AllPortsSameDT=off  OutDataTypeStr=boolean
  Logical Operator12 : Logic  AllPortsSameDT=off  OutDataTypeStr=boolean
  Logical Operator2 : Logic  Operator=OR  AllPortsSameDT=off  OutDataTypeStr=boolean
  Logical Operator7 : Logic  Operator=NOT  AllPortsSameDT=off  OutDataTypeStr=boolean
  Logical Operator8 : Logic  AllPortsSameDT=off  OutDataTypeStr=boolean
  Logical Operator9 : Logic  AllPortsSameDT=off  OutDataTypeStr=boolean
  Mux : Mux  Inputs=8
  Mux1 : Mux  Inputs=8
  Mux2 : Mux  Inputs=3
  Unit Delay : UnitDelay  SampleTime=-1
  Unit Delay1 : UnitDelay  SampleTime=-1
  bitwise_faults : Subsystem
  bitwise_status : Subsystem
  tag scope: prot=scoped
  wires:
  Data Type Conversion7/1 -> Mux/8  "ext_fault"
  ext_flt/1 -> Data Type Conversion7/1
  Unit Delay1/1 -> Bus Creator/3  "status"
  Bus Selector14/1 -> Mux2/3  "<Logic_trip>"
  Bus Selector12/1 -> Bus Selector14/1  "<cb_ctrl>"
  [logic] -> Bus Selector12/1
  [trip] -> Mux2/2
  Bus Selector10/1 -> Mux2/1  "<Enable>"
  [modbus_in] -> Bus Selector10/1
  Mux2/1 -> bitwise_status/1(S)
  [flt_latch] -> bitwise_faults/1(S)
  bitwise_faults/1(s) -> Bus Creator/4  "flt_word"
  bitwise_status/1(s) -> Unit Delay1/1
  Detect Change/1 -> Logical Operator1/3
  [flt] -> Fault_Latch/1(fault)
  Mux/1 -> [flt]
  Detect Increase2/1 -> Logical Operator2/1
  [reset] -> Detect Increase2/1
  [auto_reset] -> Logical Operator2/2
  Logical Operator2/1 -> Fault_Latch/3(reset)
  Bus Selector1/1 -> Discrete-Time Integrator1/3, Detect Change/1  "<Auto_Reset>"
  [modbus_in] -> Bus Selector1/1
  Unit Delay/1 -> [auto_reset]
  Detect Increase/1 -> Unit Delay/1
  Logical Operator1/1 -> Discrete-Time Integrator1/2
  [auto_reset] -> Logical Operator1/1
  Detect Increase1/1 -> Logical Operator1/2
  Compare To Constant/1 -> Detect Increase/1
  Discrete-Time Integrator1/1 -> Compare To Constant/1
  [trip] -> Detect Increase1/1
  Constant/1 -> Discrete-Time Integrator1/1
  Bus Creator/1 -> [prot]
  Logical Operator/1 -> [trip], Bus Creator/2  "trip"
  Data Type Conversion6/1 -> Extract Bits1/1, Extract Bits2/1, Extract Bits4/1, Extract Bits3/1
  Data Type Conversion5/1 -> Mux/4  "59"
  Data Type Conversion4/1 -> Mux/3  "27"
  Data Type Conversion2/1 -> Mux/2  "51"
  Data Type Conversion3/1 -> Mux/1  "50"
  Data Type Conversion1/1 -> Mux/7
  Data Type Conversion/1 -> Mux/6
  Fault_Latch/1(latched) -> Bus Creator/1, [flt_latch], Logical Operator/1  "flt_latched"
  Bus Selector19/3 -> [reset]  "<Reset>"
  [mask] -> Fault_Latch/4(mask)
  Logical Operator12/1 -> Mux1/7
  Logical Operator9/1 -> Mux1/6
  Logical Operator8/1 -> Mux1/5
  Logical Operator7/1 -> Logical Operator8/2
  Bus Selector19/2 -> Logical Operator7/1, Logical Operator9/2, Logical Operator12/2  "<Use_VF_Cmd>"
  Bus Selector19/1 -> Mux1/1, Mux1/4, Logical Operator8/1, Logical Operator9/1, Mux1/8, Logical Operator12/1, Mux1/3, Mux1/2  "<Enable>"
  [modbus_in] -> Bus Selector19/1
  Mux1/1 -> [mask]
  Extract Bits4/1 -> Data Type Conversion5/1
  Extract Bits3/1 -> Data Type Conversion4/1
  Extract Bits2/1 -> Data Type Conversion2/1
  Extract Bits1/1 -> Data Type Conversion3/1
  Bus Selector13/1 -> Data Type Conversion1/1  "<BattEmpty>"
  [battery] -> Bus Selector13/1
  Bus Selector11/1 -> Data Type Conversion/1  "<BattFull>"
  [battery] -> Bus Selector11/1
  Bus Selector8/1 -> Logical Operator11/1  "<lock>"
  [pll] -> Bus Selector8/1
  Logical Operator11/1 -> Mux/5
  Bus Selector6/1 -> Data Type Conversion6/1  "<status>"
  Bus Selector5/1 -> Bus Selector6/1  "<m>"
  Bus Selector4/1 -> Bus Selector5/1  "<relay_out>"
  [cb_meas] -> Bus Selector4/1
  [modbus_in] -> Bus Selector2/1
  Bus Selector2/1 -> Fault_Latch/2(enable)  "<Enable>"

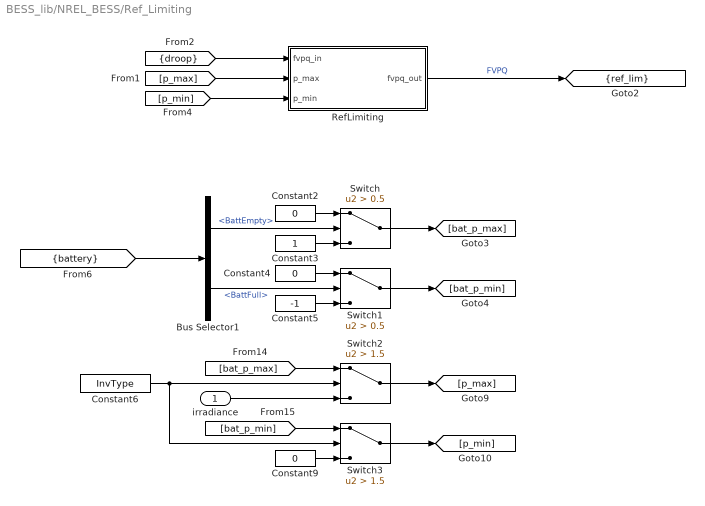
== system BESS_lib/NREL_BESS/Ref_Limiting ==
  irradiance : Inport
  Bus Selector1 : BusSelector  OutputSignals=BattEmpty,BattFull
  Constant2 : Constant  Value=0
  Constant3 : Constant
  Constant4 : Constant  Value=0
  Constant5 : Constant  Value=-1
  Constant6 : Constant  Value=InvType
  Constant9 : Constant  Value=0
  RefLimiting : Subsystem
  Switch : Switch  Criteria=u2 > Threshold  Threshold=0.5
  Switch1 : Switch  Criteria=u2 > Threshold  Threshold=0.5
  Switch2 : Switch  Criteria=u2 > Threshold  Threshold=1.5
  Switch3 : Switch  Criteria=u2 > Threshold  Threshold=1.5
  tag scope: ref_lim=scoped
  wires:
  [droop] -> RefLimiting/1(fvpq_in)
  Constant9/1 -> Switch3/3
  [bat_p_max] -> Switch2/1
  [bat_p_min] -> Switch3/1
  irradiance/1 -> Switch2/3
  Constant6/1 -> Switch2/2, Switch3/2
  Switch2/1 -> [p_max]
  Switch3/1 -> [p_min]
  [p_max] -> RefLimiting/2(p_max)
  [p_min] -> RefLimiting/3(p_min)
  Bus Selector1/1 -> Switch/2  "<BattEmpty>"
  Switch/1 -> [bat_p_max]
  Switch1/1 -> [bat_p_min]
  Bus Selector1/2 -> Switch1/2  "<BattFull>"
  Constant2/1 -> Switch/1
  Constant3/1 -> Switch/3
  Constant4/1 -> Switch1/1
  Constant5/1 -> Switch1/3
  [battery] -> Bus Selector1/1
  RefLimiting/1(fvpq_out) -> [ref_lim]  "FVPQ"

== system BESS_lib/NREL_BESS/Battery/Battery ==
  note: wHr/s
  note: wHr
  Iout : Inport
  cap_div : Inport  Port=2
  soc_rst : Inport  Port=3
  Add : Sum  Inputs=+-
  Constant : Constant  Value=Vdc_nom
  Discrete-Time Integrator : DiscreteIntegrator  ExternalReset=level  InitialCondition=kWh*0.8*1000  InitialConditionMode=State only (most efficient)  SampleTime=-1  LimitOutput=on  UpperSaturationLimit=kWh*1000  LowerSaturationLimit=0  ShowSaturationPort=on  ICPrevOutput=DiscIntNeverNeededParam  ICPrevScaledInput=DiscIntNeverNeededParam
  Gain1 : Gain  Gain=-Vdc_nom/3600
  Gain2 : Gain  Gain=1/(kWh*1000)
  IC1 : InitialCondition  Value=Vdc_nom
  Memory : Memory
  Product : Product
  Resr : Gain  Gain=esr
  Vout : Outport
  Capacity : Outport  Port=2
  Saturation : Outport  Port=3
  wires:
  cap_div/1 -> Product/1
  soc_rst/1 -> Discrete-Time Integrator/2
  Gain1/1 -> Discrete-Time Integrator/1
  Memory/1 -> IC1/1
  Iout/1 -> Resr/1, Product/2
  Gain2/1 -> Capacity/1
  Discrete-Time Integrator/1 -> Gain2/1
  IC1/1 -> Vout/1
  Product/1 -> Gain1/1
  Discrete-Time Integrator/2 -> Saturation/1
  Constant/1 -> Add/1
  Resr/1 -> Add/2
  Add/1 -> Memory/1

== system BESS_lib/NREL_BESS/Droop/Droop ==
  dfvpq : Inport
  droop : Inport  Port=2
  Demux : Demux
  Demux1 : Demux
  Low Pass{1..4} (4 alike) : DiscreteStateSpace  A=BP.filt.A  B=BP.filt.B  C=BP.filt.C  D=BP.filt.D  SampleTime=-1
  Mux1 : Mux
  Product{,1..3} (4 alike) : Product
  Selector : Selector  InputPortWidth=4  IndexOptions=Index vector (dialog)  Indices=[3 4 1 2]  OutputSizes=1
  dFvpq_out : Outport
  wires:
  Demux/3 -> Low Pass3/1  "p"
  Low Pass2/1 -> Product1/1
  Demux/2 -> Low Pass1/1  "v"
  Demux/1 -> Low Pass2/1  "f"
  Low Pass3/1 -> Product/1
  dfvpq/1 -> Demux/1
  Selector/1 -> dFvpq_out/1
  Low Pass1/1 -> Product3/1
  Demux/4 -> Low Pass4/1  "q"
  Low Pass4/1 -> Product2/1
  Product1/1 -> Mux1/1  "p"
  Product3/1 -> Mux1/2  "q"
  Product/1 -> Mux1/3  "F"
  Product2/1 -> Mux1/4  "v"
  Mux1/1 -> Selector/1
  Demux1/1 -> Product1/2
  Demux1/4 -> Product2/2
  Demux1/3 -> Product/2
  Demux1/2 -> Product3/2
  droop/1 -> Demux1/1

== system BESS_lib/NREL_BESS/Droop/ExtractCoefs ==
  In1 : Inport
  Bus Selector8 : BusSelector  OutputSignals=FP_droop,VQ_droop,FP_droop,VQ_droop
  Mux : Mux
  Out1 : Outport
  wires:
  Bus Selector8/1 -> Mux/1  "<FP_droop>"
  Bus Selector8/4 -> Mux/4  "<VQ_droop>"
  Bus Selector8/2 -> Mux/2  "<VQ_droop>"
  Bus Selector8/3 -> Mux/3  "<FP_droop>"
  Mux/1 -> Out1/1
  In1/1 -> Bus Selector8/1

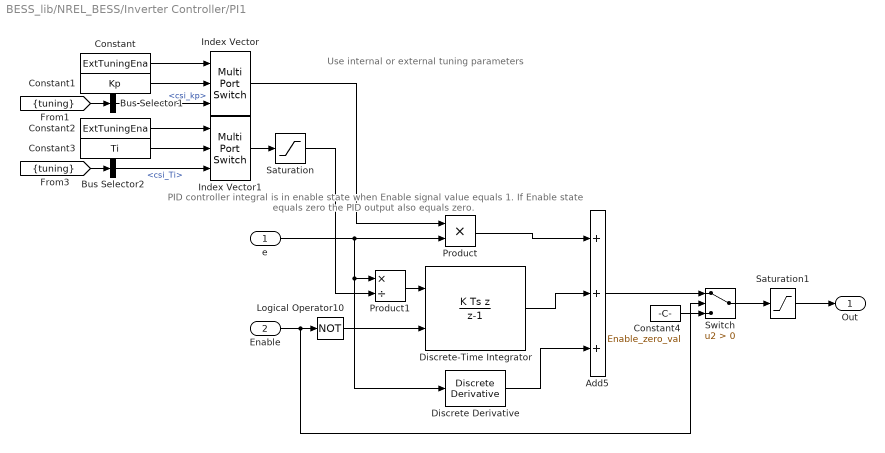
== system BESS_lib/NREL_BESS/Inverter Controller/PI1 ==
  note: PID controller integral is in enable state when Enable signal value equals 1. If Enable state equals zero the PID output also equals zero.
  note: Use internal or external tuning parameters
  e : Inport
  Enable : Inport  Port=2
  Add5 : Sum  Inputs=+++
  Bus Selector1 : BusSelector  OutputSignals=csi_kp
  Bus Selector2 : BusSelector  OutputSignals=csi_Ti
  Constant : Constant  Value=ExtTuningEna
  Constant1 : Constant  Value=Kp
  Constant2 : Constant  Value=ExtTuningEna
  Constant3 : Constant  Value=Ti
  Constant4 : Constant  Value=Enable_zero_val
  Discrete Derivative : simulink/Discrete/Discrete Derivative  gainval=D  ICPrevScaledInput=0.0  InputProcessing=Inherited  OutMin=[]  OutMax=[]  OutDataType=fixdt(1, 16)  OutScaling=2^-10  DoSatur=off
  Discrete-Time Integrator : DiscreteIntegrator  IntegratorMethod=Integration: Backward Euler  gainval=1  ExternalReset=level  InitialCondition=Int_init  SampleTime=Ts  LimitOutput=on  UpperSaturationLimit=Iup  LowerSaturationLimit=Idown  ICPrevOutput=DiscIntNeverNeededParam  ICPrevScaledInput=DiscIntNeverNeededParam
  Index Vector : MultiPortSwitch  DataPortOrder=Zero-based contiguous  Inputs=2  zeroidx=on
  Index Vector1 : MultiPortSwitch  DataPortOrder=Zero-based contiguous  Inputs=2  zeroidx=on
  Logical Operator10 : Logic  Operator=NOT  IconShape=distinctive  AllPortsSameDT=off  OutDataTypeStr=boolean
  Product : Product
  Product1 : Product  Inputs=*/
  Saturation : Saturate  UpperLimit=inf  LowerLimit=0.0001
  Saturation1 : Saturate  UpperLimit=PIup  LowerLimit=PIdown  LinearizeAsGain=off
  Switch : Switch  Criteria=u2 > Threshold
  Out : Outport
  wires:
  Saturation/1 -> Product1/2
  Index Vector1/1 -> Saturation/1
  Product1/1 -> Discrete-Time Integrator/1
  Constant3/1 -> Index Vector1/2
  Bus Selector2/1 -> Index Vector1/3  "<csi_Ti>"
  [tuning] -> Bus Selector2/1
  Constant2/1 -> Index Vector1/1
  Index Vector/1 -> Product/1
  Constant1/1 -> Index Vector/2
  Bus Selector1/1 -> Index Vector/3  "<csi_kp>"
  [tuning] -> Bus Selector1/1
  Constant/1 -> Index Vector/1
  Discrete Derivative/1 -> Add5/3
  Add5/1 -> Switch/1
  Constant4/1 -> Switch/3
  Logical Operator10/1 -> Discrete-Time Integrator/2
  e/1 -> Product1/1, Discrete Derivative/1, Product/2
  Discrete-Time Integrator/1 -> Add5/2
  Product/1 -> Add5/1
  Enable/1 -> Switch/2, Logical Operator10/1
  Switch/1 -> Saturation1/1
  Saturation1/1 -> Out/1

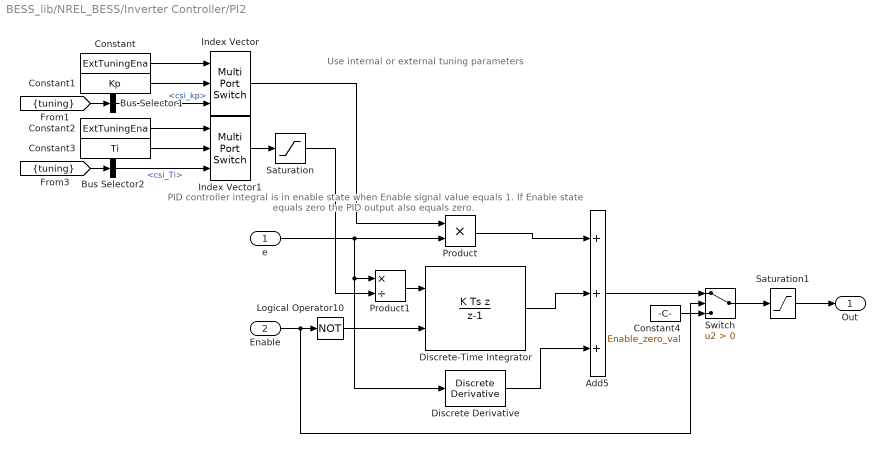
== system BESS_lib/NREL_BESS/Inverter Controller/PI2 ==
  note: Use internal or external tuning parameters
  note: PID controller integral is in enable state when Enable signal value equals 1. If Enable state equals zero the PID output also equals zero.
  e : Inport
  Enable : Inport  Port=2
  Add5 : Sum  Inputs=+++
  Bus Selector1 : BusSelector  OutputSignals=csi_kp
  Bus Selector2 : BusSelector  OutputSignals=csi_Ti
  Constant : Constant  Value=ExtTuningEna
  Constant1 : Constant  Value=Kp
  Constant2 : Constant  Value=ExtTuningEna
  Constant3 : Constant  Value=Ti
  Constant4 : Constant  Value=Enable_zero_val
  Discrete Derivative : simulink/Discrete/Discrete Derivative  gainval=D  ICPrevScaledInput=0.0  InputProcessing=Inherited  OutMin=[]  OutMax=[]  OutDataType=fixdt(1, 16)  OutScaling=2^-10  DoSatur=off
  Discrete-Time Integrator : DiscreteIntegrator  IntegratorMethod=Integration: Backward Euler  gainval=1  ExternalReset=level  InitialCondition=Int_init  SampleTime=Ts  LimitOutput=on  UpperSaturationLimit=Iup  LowerSaturationLimit=Idown  ICPrevOutput=DiscIntNeverNeededParam  ICPrevScaledInput=DiscIntNeverNeededParam
  Index Vector : MultiPortSwitch  DataPortOrder=Zero-based contiguous  Inputs=2  zeroidx=on
  Index Vector1 : MultiPortSwitch  DataPortOrder=Zero-based contiguous  Inputs=2  zeroidx=on
  Logical Operator10 : Logic  Operator=NOT  IconShape=distinctive  AllPortsSameDT=off  OutDataTypeStr=boolean
  Product : Product
  Product1 : Product  Inputs=*/
  Saturation : Saturate  UpperLimit=inf  LowerLimit=0.0001
  Saturation1 : Saturate  UpperLimit=PIup  LowerLimit=PIdown  LinearizeAsGain=off
  Switch : Switch  Criteria=u2 > Threshold
  Out : Outport
  wires:
  Saturation1/1 -> Out/1
  Switch/1 -> Saturation1/1
  Enable/1 -> Logical Operator10/1, Switch/2
  Product/1 -> Add5/1
  Discrete-Time Integrator/1 -> Add5/2
  e/1 -> Product/2, Discrete Derivative/1, Product1/1
  Logical Operator10/1 -> Discrete-Time Integrator/2
  Constant4/1 -> Switch/3
  Add5/1 -> Switch/1
  Discrete Derivative/1 -> Add5/3
  Constant/1 -> Index Vector/1
  [tuning] -> Bus Selector1/1
  Bus Selector1/1 -> Index Vector/3  "<csi_kp>"
  Constant1/1 -> Index Vector/2
  Index Vector/1 -> Product/1
  Constant2/1 -> Index Vector1/1
  [tuning] -> Bus Selector2/1
  Bus Selector2/1 -> Index Vector1/3  "<csi_Ti>"
  Constant3/1 -> Index Vector1/2
  Product1/1 -> Discrete-Time Integrator/1
  Index Vector1/1 -> Saturation/1
  Saturation/1 -> Product1/2

== system BESS_lib/NREL_BESS/Inverter Controller/rate_limit ==
  in : Inport
  rst : Inport  Port=2
  Demux : Demux  Outputs=2
  Mux : Mux  Inputs=2
  RateLimitwRst : Subsystem
  RateLimitwRst1 : Subsystem
  out : Outport
  wires:
  rst/1 -> RateLimitwRst1/1(Rst), RateLimitwRst/1(Rst)
  RateLimitwRst1/1(Out) -> Mux/2
  Demux/1 -> RateLimitwRst/2(In)
  in/1 -> Demux/1
  RateLimitwRst/1(Out) -> Mux/1
  Demux/2 -> RateLimitwRst1/2(In)
  Mux/1 -> out/1  "fvpq"

== system BESS_lib/NREL_BESS/PLL/PLL (3ph)1 ==
  abc : Inport  PortDimensions=3  SampleTime=Ts
  Model : Subsystem  DialogController=POWERSYS.PowerSysDialog
  Freq : Outport  SampleTime=Ts
  wt : Outport  Port=2  SampleTime=Ts
  Lock : Outport  Port=3  SampleTime=Ts
  wires:
  Model/2(wt) -> wt/1
  Model/1(Freq) -> Freq/1
  abc/1 -> Model/1(Vabc)
  Model/3(Lock) -> Lock/1

== system BESS_lib/NREL_BESS/PLL/VCO ==
  w : Inport
  rst : Inport  Port=2
  init : Inport  Port=3
  Compare To Constant : simulink/Logic and Bit Operations/Compare To Constant  relop=>=  const=pi  OutDataTypeStr=uint8
  Gain : Gain  Gain=2*pi  OutDataTypeStr=double
  Gain2 : Gain  Gain=Ts  SaturateOnIntegerOverflow=on  OutDataTypeStr=Inherit: Same as input  ParamDataTypeStr=Inherit: Same as input
  Sum : Sum  Inputs=-++
  Switch : Switch  Threshold=0.5
  Unit Delay1 : UnitDelay  SampleTime=-1
  theta : Outport
  wires:
  init/1 -> Switch/1
  rst/1 -> Switch/2
  Switch/1 -> Unit Delay1/1
  Sum/1 -> Switch/3
  Gain2/1 -> Sum/2
  Unit Delay1/1 -> Compare To Constant/1, theta/1, Sum/3  "wt"
  Compare To Constant/1 -> Gain/1
  Gain/1 -> Sum/1
  w/1 -> Gain2/1

== system BESS_lib/NREL_BESS/Protection/Fault_Latch ==
  fault : Inport
  enable : Inport  Port=2
  reset : Inport  Port=3
  mask : Inport  Port=4
  Logical Operator1 : Logic  Operator=OR  AllPortsSameDT=off  OutDataTypeStr=boolean
  Logical Operator2 : Logic  Operator=NOT  AllPortsSameDT=off  OutDataTypeStr=boolean
  Logical Operator6 : Logic  Inputs=3  AllPortsSameDT=off  OutDataTypeStr=boolean
  SR_Prior_S : Subsystem
  latched : Outport
  wires:
  SR_Prior_S/1(Q) -> latched/1
  Logical Operator6/1 -> SR_Prior_S/1(S)
  [reset] -> Logical Operator1/1
  reset/1 -> [reset]
  [ena] -> Logical Operator6/3
  enable/1 -> [ena]
  fault/1 -> Logical Operator6/1
  mask/1 -> [mask]
  [mask] -> Logical Operator6/2
  [mask] -> Logical Operator2/1
  Logical Operator1/1 -> SR_Prior_S/2(R)
  Logical Operator2/1 -> Logical Operator1/2
